simulink library "J2000toGeoc"  (R2014b)
settings: Solver=ode45  StartTime=0.0  StopTime=10.0  RelTol=1e-3
undefined symbols (not defined in the file): ConfParam
settings Model: Creator=Hp  LastModifiedBy=Hp

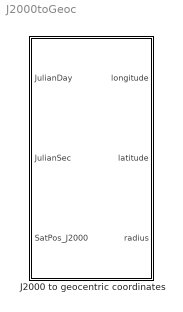
== system J2000toGeoc ==
  J2000 to geocentric coordinates : Subsystem

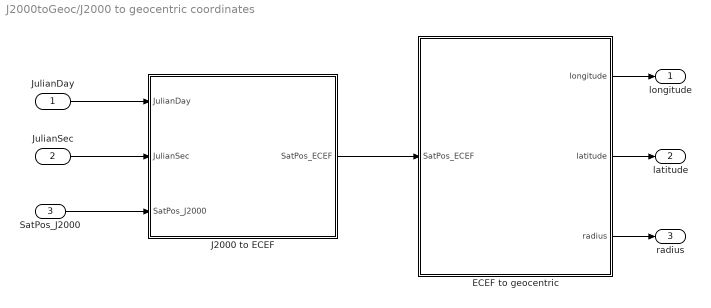
== system J2000toGeoc/J2000 to geocentric coordinates ==
  JulianDay : Inport
  JulianSec : Inport  Port=2
  SatPos_J2000 : Inport  Port=3
  ECEF to geocentric : Subsystem
  J2000 to ECEF : Subsystem
  longitude : Outport
  latitude : Outport  Port=2
  radius : Outport  Port=3
  wires:
  J2000 to ECEF/1(SatPos_ECEF) -> ECEF to geocentric/1(SatPos_ECEF)
  SatPos_J2000/1 -> J2000 to ECEF/3(SatPos_J2000)
  JulianSec/1 -> J2000 to ECEF/2(JulianSec)
  JulianDay/1 -> J2000 to ECEF/1(JulianDay)
  ECEF to geocentric/2(latitude) -> latitude/1
  ECEF to geocentric/3(radius) -> radius/1
  ECEF to geocentric/1(longitude) -> longitude/1

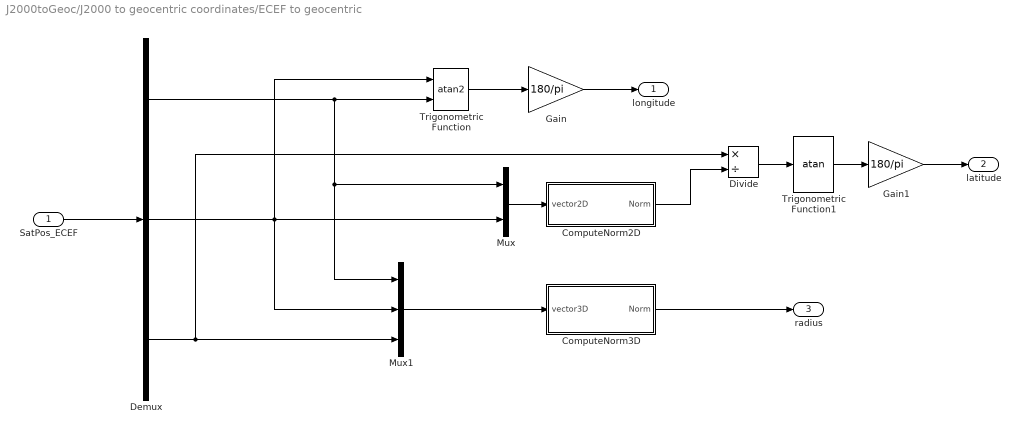
== system J2000toGeoc/J2000 to geocentric coordinates/ECEF to geocentric ==
  SatPos_ECEF : Inport
  ComputeNorm2D : Subsystem
  ComputeNorm3D : Subsystem
  Demux : Demux  Outputs=3
  Divide : Product  Inputs=*/
  Gain : Gain  Gain=180/pi
  Gain1 : Gain  Gain=180/pi
  Mux : Mux  Inputs=2
  Mux1 : Mux  Inputs=3
  Trigonometric Function : Trigonometry  Operator=atan2
  Trigonometric Function1 : Trigonometry  Operator=atan
  longitude : Outport
  latitude : Outport  Port=2
  radius : Outport  Port=3
  wires:
  SatPos_ECEF/1 -> Demux/1
  Demux/1 -> Mux/1, Mux1/1, Trigonometric Function/2
  Demux/2 -> Trigonometric Function/1, Mux/2, Mux1/2
  Demux/3 -> Divide/1, Mux1/3
  Trigonometric Function/1 -> Gain/1
  Gain/1 -> longitude/1
  Divide/1 -> Trigonometric Function1/1
  ComputeNorm2D/1(Norm) -> Divide/2
  Mux1/1 -> ComputeNorm3D/1(vector3D)
  ComputeNorm3D/1(Norm) -> radius/1
  Mux/1 -> ComputeNorm2D/1(vector2D)
  Trigonometric Function1/1 -> Gain1/1
  Gain1/1 -> latitude/1

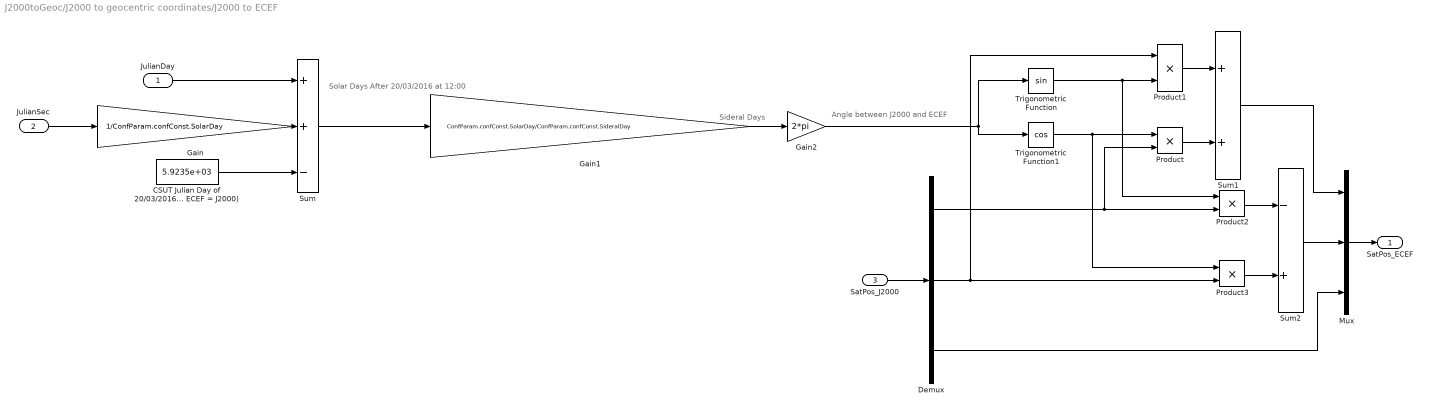
== system J2000toGeoc/J2000 to geocentric coordinates/J2000 to ECEF ==
  note: Solar Days After 20/03/2016 at 12:00
  note: Sideral Days
  note: Angle between J2000 and ECEF
  JulianDay : Inport
  JulianSec : Inport  Port=2
  SatPos_J2000 : Inport  Port=3
  CSUT Julian Day of 20/03/2016 at 12:00 UTC (moment in which ECEF = J2000) : Constant  Value=5.9235e+03
  Demux : Demux  Outputs=3
  Gain : Gain  Gain=1/ConfParam.confConst.SolarDay
  Gain1 : Gain  Gain=ConfParam.confConst.SolarDay/ConfParam.confConst.SideralDay
  Gain2 : Gain  Gain=2*pi
  Mux : Mux  Inputs=3
  Product{,1..3} (4 alike) : Product
  Sum : Sum  Inputs=++-
  Sum1 : Sum
  Sum2 : Sum  Inputs=-+
  Trigonometric Function : Trigonometry
  Trigonometric Function1 : Trigonometry  Operator=cos
  SatPos_ECEF : Outport
  wires:
  Trigonometric Function/1 -> Product1/2, Product2/1
  Gain1/1 -> Gain2/1
  Gain2/1 -> Trigonometric Function/1, Trigonometric Function1/1
  Sum/1 -> Gain1/1
  Gain/1 -> Sum/2
  Trigonometric Function1/1 -> Product/1, Product3/1
  Demux/3 -> Mux/3
  Sum2/1 -> Mux/2
  Product3/1 -> Sum2/2
  Product/1 -> Sum1/2
  Demux/1 -> Product2/2, Product/2
  Demux/2 -> Product1/1, Product3/2
  Product2/1 -> Sum2/1
  SatPos_J2000/1 -> Demux/1
  CSUT Julian Day of 20/03/2016 at 12:00 UTC (moment in which ECEF = J2000)/1 -> Sum/3
  Product1/1 -> Sum1/1
  JulianSec/1 -> Gain/1
  Sum1/1 -> Mux/1
  JulianDay/1 -> Sum/1
  Mux/1 -> SatPos_ECEF/1

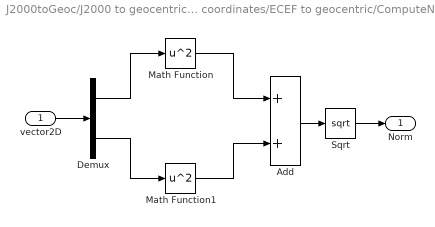
== system J2000toGeoc/J2000 to geocentric coordinates/ECEF to geocentric/ComputeNorm2D ==
  vector2D : Inport
  Add : Sum
  Demux : Demux  Outputs=2
  Math Function : Math  Operator=square  SaturateOnIntegerOverflow=on
  Math Function1 : Math  Operator=square  SaturateOnIntegerOverflow=on
  Sqrt : Sqrt  SaturateOnIntegerOverflow=on
  Norm : Outport
  wires:
  Demux/2 -> Math Function1/1
  Math Function/1 -> Add/1
  Demux/1 -> Math Function/1
  Math Function1/1 -> Add/2
  Add/1 -> Sqrt/1
  Sqrt/1 -> Norm/1
  vector2D/1 -> Demux/1

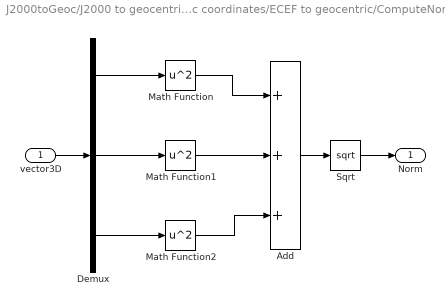
== system J2000toGeoc/J2000 to geocentric coordinates/ECEF to geocentric/ComputeNorm3D ==
  vector3D : Inport
  Add : Sum  Inputs=+++
  Demux : Demux  Outputs=3
  Math Function : Math  Operator=square  SaturateOnIntegerOverflow=on
  Math Function1 : Math  Operator=square  SaturateOnIntegerOverflow=on
  Math Function2 : Math  Operator=square  SaturateOnIntegerOverflow=on
  Sqrt : Sqrt  SaturateOnIntegerOverflow=on
  Norm : Outport
  wires:
  Demux/2 -> Math Function1/1
  Demux/3 -> Math Function2/1
  Math Function/1 -> Add/1
  Demux/1 -> Math Function/1
  Math Function2/1 -> Add/3
  Math Function1/1 -> Add/2
  Add/1 -> Sqrt/1
  Sqrt/1 -> Norm/1
  vector3D/1 -> Demux/1
